simulink model "position_control_PD_with_Due"  (R2022a)
settings: Solver=FixedStepAuto  StartTime=0.0  StopTime=6  FixedStep=0.01  RelTol=1e-3  EnableMultiTasking=on
undefined symbols (not defined in the file or in its folder): a, b, kd2, kd4, kp2, kp4
libraries: arduinolib x11, arduinosensorlib x4
settings Model: SimulationMode=external  ExtModeTrigDuration=2  Creator=DCLab  LastModifiedBy=LabPC
settings OptimizationCC: EnhancedBackFolding=on  PassReuseOutputArgsAs=Individual arguments  ZeroExternalMemoryAtStartup=off  ZeroInternalMemoryAtStartup=off  MaxStackSize=64  OptimizeBlockOrder=speed  DifferentSizesBufferReuse=on  OptimizationCustomize=off  EfficientTunableParamExpr=on
settings DebuggingCC: ParameterTunabilityLossMsg=error  UnconnectedInputMsg=warning  UnconnectedOutputMsg=warning  UnconnectedLineMsg=warning
settings HardwareCC: ProdBitPerInt=16  ProdBitPerPointer=16  ProdBitPerSizeT=16  ProdBitPerPtrDiffT=16  ProdLargestAtomicFloat=None  ProdWordSize=8  ProdHWDeviceType=Atmel->AVR
settings SFSimCC: MATLABDynamicMemAlloc=off  SimTargetLang=C++
settings RTWCC: SystemTargetFile=ert.tlc  HardwareBoard=Arduino Uno  TemplateMakefile=ert_default_tmf  Toolchain=Arduino AVR  BuildConfiguration=Faster Runs  DLArmComputeVersion=19.05
settings CodeAppCC: ForceParamTrailComments=on  IgnoreCustomStorageClasses=off  OperatorAnnotations=on  SimulinkDataObjDesc=on  SFDataObjDesc=on  InsertBlockDesc=on
settings ERTTargetCC: SupportContinuousTime=on  SupportVariableSizeSignals=on  ExtMode=on  ExtModeTransport=3  ExtModeStaticAlloc=on  ExtModeStaticAllocSize=250  ExtModeMexFile=ext_xcp  ExtModeMexArgs=0 3 115200  ExtModeIntrfLevel=Level2 - Open

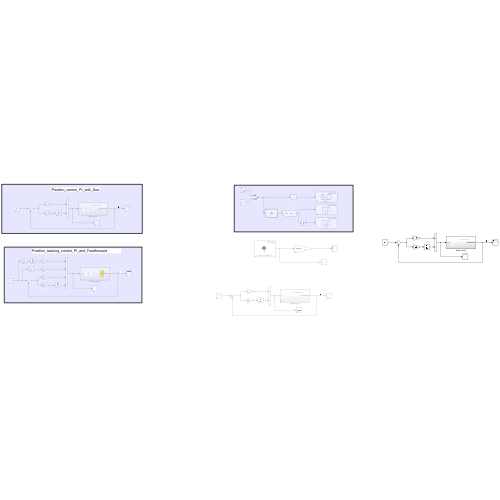
[thumbnail: Simulink's stored preview of the top-level diagram]
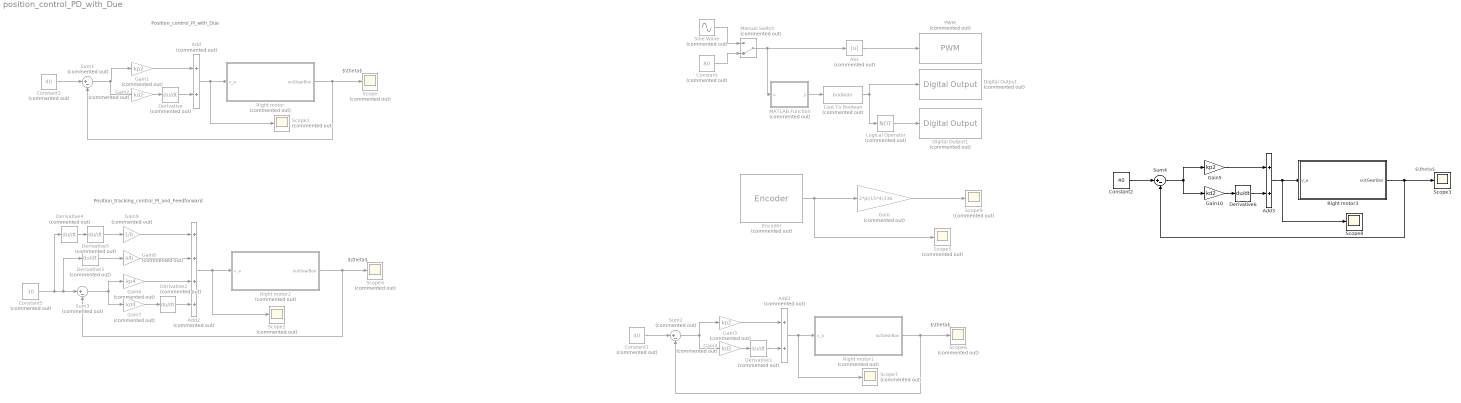
== system position_control_PD_with_Due ==
  note: Position_control_PI_with_Due
  note: $\theta$
  note: $\theta$
  note: Position_tracking_control_PI_and_Feedforward
  note: $\theta$
  note: $\theta$
  Abs : Abs  Commented=on  SaturateOnIntegerOverflow=off
  Add : Sum  Commented=on
  Add1 : Sum  Commented=on
  Add2 : Sum  Commented=on  Inputs=++++
  Add3 : Sum
  Cast To Boolean : DataTypeConversion  Commented=on  OutDataTypeStr=boolean  SaturateOnIntegerOverflow=off  RndMeth=Floor
  Constant : Constant  Commented=on  Value=80
  Constant1 : Constant  Commented=on  Value=40
  Constant2 : Constant  Value=40
  Constant3 : Constant  Commented=on  Value=40
  Constant5 : Constant  Commented=on  Value=30
  Derivative{,1..5} (6 alike) : Derivative  Commented=on
  Derivative6 : Derivative
  Digital Output : arduinolib/Digital Output  Commented=on  pinNumber=6  Direction=output  blockPlatform=arduino
  Digital Output1 : arduinolib/Digital Output  Commented=on  pinNumber=7  Direction=output  blockPlatform=arduino
  Encoder : arduinosensorlib/Encoder  Commented=on  InputA=2  InputB=3  Mode=Reset at each Sample time  SampleTime=-1
      settings: SourceProductBaseCode=ARDUINO
  Gain : Gain  Commented=on  Gain=2*pi/15*4/336
  Gain1 : Gain  Commented=on  Gain=kp2
  Gain10 : Gain  Gain=kd2
  Gain2 : Gain  Commented=on  Gain=kd2
  Gain3 : Gain  Commented=on  Gain=kp2
  Gain4 : Gain  Commented=on  Gain=kd2
  Gain5 : Gain  Gain=kp2
  Gain6 : Gain  Commented=on  Gain=kp4
  Gain7 : Gain  Commented=on  Gain=kd4
  Gain8 : Gain  Commented=on  Gain=a/b
  Gain9 : Gain  Commented=on  Gain=1/b
  Logical Operator : Logic  Commented=on  Operator=NOT  AllPortsSameDT=off  OutDataTypeStr=boolean
  MATLAB Function : MATLAB Function  Commented=on  TreatAsAtomicUnit=on
  Manual Switch : ManualSwitch  Commented=on  CurrentSetting=0
  PWM : arduinolib/PWM  Commented=on  pinNumber=5  frequencyType=Default  desiredFrequency=490.2  achievableFrequency=490.2
  Right motor : Subsystem  Commented=on
  Right motor1 : Subsystem  Commented=on
  Right motor2 : Subsystem  Commented=on
  Right motor3 : Subsystem
  Scope{,1..2,4..7,9} (8 alike) : Scope  Commented=on
  Scope3 : Scope
  Scope8 : Scope
  Sine Wave : Sin  Commented=on  Amplitude=255  SampleTime=0
  Sum1 : Sum  Commented=on  Inputs=|+-
  Sum2 : Sum  Commented=on  Inputs=|+-
  Sum3 : Sum  Commented=on  Inputs=|+-
  Sum4 : Sum  Inputs=|+-
  wires:
  Gain2/1 -> Derivative/1
  Sum1/1 -> Gain2/1, Gain1/1
  Derivative/1 -> Add/2
  Gain1/1 -> Add/1
  Add/1 -> Scope1/1, Right motor/1(v_a)
  Right motor/1(outGearBox) -> Sum1/2, Scope/1
  Constant3/1 -> Sum1/1
  Sum3/1 -> Gain6/1, Gain7/1
  Gain9/1 -> Add2/1
  Derivative2/1 -> Add2/4
  Gain6/1 -> Add2/3
  Constant5/1 -> Derivative4/1, Derivative3/1, Sum3/1
  Gain7/1 -> Derivative2/1
  Gain8/1 -> Add2/2
  Derivative3/1 -> Gain8/1
  Derivative4/1 -> Derivative5/1
  Derivative5/1 -> Gain9/1
  Right motor2/1(outGearBox) -> Sum3/2, Scope4/1
  Add2/1 -> Scope2/1, Right motor2/1(v_a)
  MATLAB Function/1(y) -> Cast To Boolean/1
  Cast To Boolean/1 -> Logical Operator/1, Digital Output/1
  Logical Operator/1 -> Digital Output1/1
  Abs/1 -> PWM/1
  Encoder/1 -> Scope5/1, Gain/1
  Sine Wave/1 -> Manual Switch/1
  Manual Switch/1 -> MATLAB Function/1(u), Abs/1
  Constant/1 -> Manual Switch/2
  Constant1/1 -> Sum2/1
  Right motor1/1(outGearBox) -> Scope6/1, Sum2/2
  Add1/1 -> Right motor1/1(v_a), Scope7/1
  Gain3/1 -> Add1/1
  Derivative1/1 -> Add1/2
  Sum2/1 -> Gain3/1, Gain4/1
  Gain4/1 -> Derivative1/1
  Constant2/1 -> Sum4/1
  Right motor3/1(outGearBox) -> Scope3/1, Sum4/2
  Add3/1 -> Right motor3/1(v_a), Scope8/1
  Gain5/1 -> Add3/1
  Derivative6/1 -> Add3/2
  Sum4/1 -> Gain5/1, Gain10/1
  Gain10/1 -> Derivative6/1
  Gain/1 -> Scope9/1

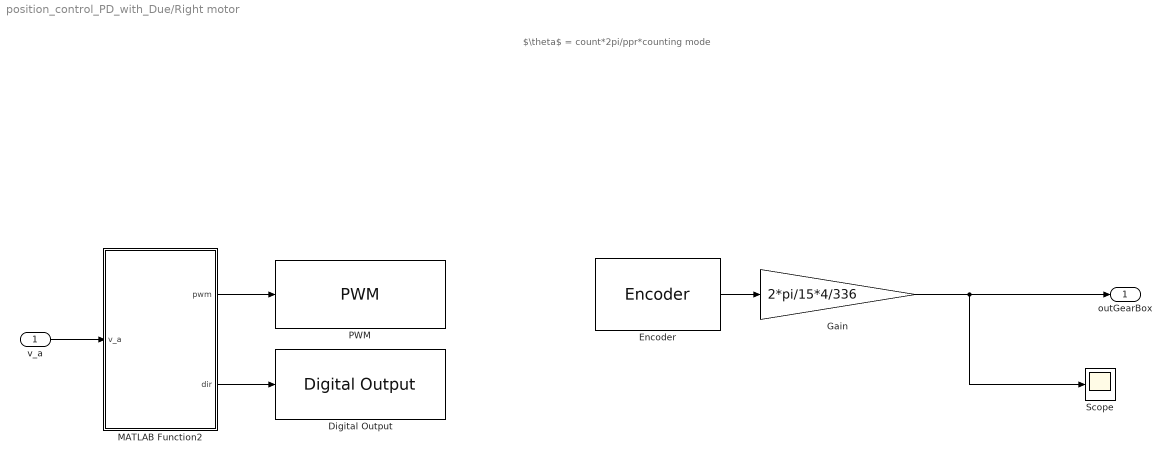
== system position_control_PD_with_Due/Right motor ==
  note: $\theta$ = count*2pi/ppr*counting mode
  v_a : Inport
  Digital Output : arduinolib/Digital Output  pinNumber=7  Direction=output  blockPlatform=arduino
  Encoder : arduinosensorlib/Encoder  InputA=2  InputB=3  Mode=No reset  SampleTime=-1
      settings: SourceProductBaseCode=ARDUINO
  Gain : Gain  Gain=2*pi/15*4/336
  MATLAB Function2 : MATLAB Function  TreatAsAtomicUnit=on
  PWM : arduinolib/PWM  pinNumber=5  frequencyType=Default  desiredFrequency=490.2  achievableFrequency=490.2
  Scope : Scope
  outGearBox : Outport
  wires:
  v_a/1 -> MATLAB Function2/1(v_a)
  MATLAB Function2/2(dir) -> Digital Output/1
  MATLAB Function2/1(pwm) -> PWM/1
  Encoder/1 -> Gain/1
  Gain/1 -> Scope/1, outGearBox/1

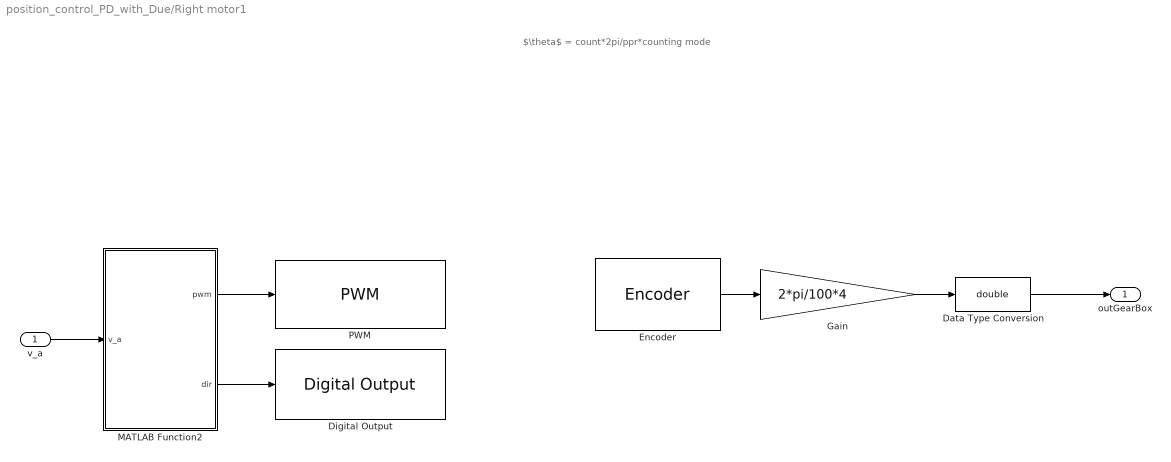
== system position_control_PD_with_Due/Right motor1 ==
  note: $\theta$ = count*2pi/ppr*counting mode
  v_a : Inport
  Data Type Conversion : DataTypeConversion  OutDataTypeStr=double  SaturateOnIntegerOverflow=off  RndMeth=Floor
  Digital Output : arduinolib/Digital Output  pinNumber=7  Direction=output  blockPlatform=arduino
  Encoder : arduinosensorlib/Encoder  InputA=2  InputB=3  Mode=No reset  SampleTime=-1
      settings: SourceProductBaseCode=ARDUINO
  Gain : Gain  Gain=2*pi/100*4
  MATLAB Function2 : MATLAB Function  TreatAsAtomicUnit=on
  PWM : arduinolib/PWM  pinNumber=6  frequencyType=Default  desiredFrequency=490.2  achievableFrequency=490.2
  outGearBox : Outport
  wires:
  Data Type Conversion/1 -> outGearBox/1
  Gain/1 -> Data Type Conversion/1
  Encoder/1 -> Gain/1
  MATLAB Function2/1(pwm) -> PWM/1
  MATLAB Function2/2(dir) -> Digital Output/1
  v_a/1 -> MATLAB Function2/1(v_a)

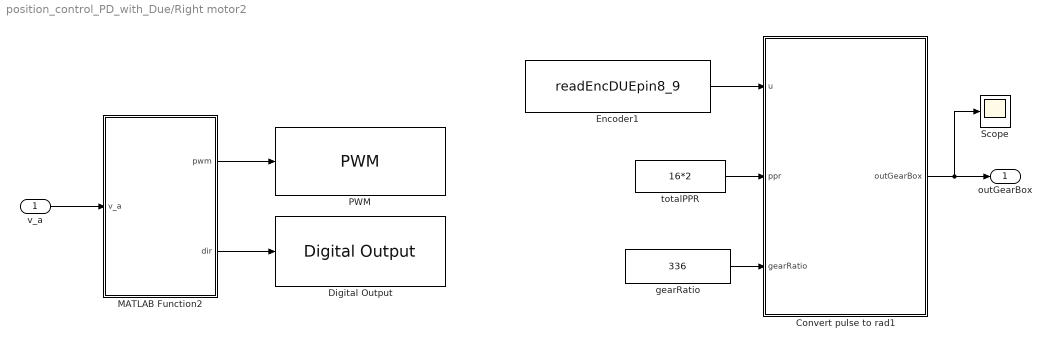
== system position_control_PD_with_Due/Right motor2 ==
  v_a : Inport
  Convert pulse to rad1 : MATLAB Function  TreatAsAtomicUnit=on
  Digital Output : arduinolib/Digital Output  pinNumber=7  Direction=output  blockPlatform=arduino
  Encoder1 : S-Function  InitFcn=try, set_param(gcb,'FunctionName','readEncDUEpin8_9'), end  FunctionName=readEncDUEpin8_9  SFunctionModules=readEncDUEpin8_9_wrapper  SFunctionDeploymentMode=off  EnableBusSupport=off  mask(S-Function Builder){}
      mask help: Simulink:masks:SFunctionBuilder_MD
      mask init:
      | val = [[.9  0.75 0.75 1 1 .9 .9 1]',[1 1 0.75 0.75 .9 .9 1 .9]'];try , sys = get_param(gcb,'SfunBuilderFcnName');if isempty(sys), sys = get_param(gcb,'FunctionName'); end,catch, sys = get_param(gcb,'FunctionName'); end
      settings: CopyFcn=set_param(gcbh,'LinkStatus','none')  PreSaveFcn=try, set_param(gcb,'FunctionName','readEncDUEpin8_9'), end  OpenFcn=sfunctionwizard(gcbh)
      mask Display:
      | plot(val(:,1),val(:,2))
      | disp(sys)
      | port_label('output',1,'count')
  MATLAB Function2 : MATLAB Function  TreatAsAtomicUnit=on
  PWM : arduinolib/PWM  pinNumber=5  frequencyType=Default  desiredFrequency=490.2  achievableFrequency=490.2
  Scope : Scope
  gearRatio : Constant  Value=336
  totalPPR : Constant  Value=16*2
  outGearBox : Outport
  wires:
  totalPPR/1 -> Convert pulse to rad1/2(ppr)
  v_a/1 -> MATLAB Function2/1(v_a)
  MATLAB Function2/2(dir) -> Digital Output/1
  MATLAB Function2/1(pwm) -> PWM/1
  gearRatio/1 -> Convert pulse to rad1/3(gearRatio)
  Convert pulse to rad1/1(outGearBox) -> Scope/1, outGearBox/1
  Encoder1/1 -> Convert pulse to rad1/1(u)

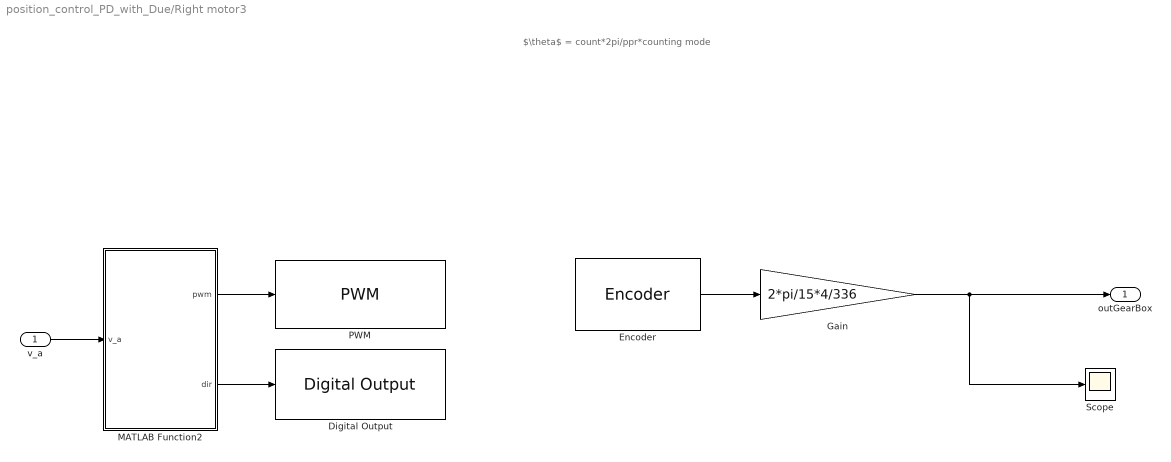
== system position_control_PD_with_Due/Right motor3 ==
  note: $\theta$ = count*2pi/ppr*counting mode
  v_a : Inport
  Digital Output : arduinolib/Digital Output  pinNumber=7  Direction=output  blockPlatform=arduino
  Encoder : arduinosensorlib/Encoder  InputA=2  InputB=3  Mode=No reset  SampleTime=-1
      settings: SourceProductBaseCode=ARDUINO
  Gain : Gain  Gain=2*pi/15*4/336
  MATLAB Function2 : MATLAB Function  TreatAsAtomicUnit=on
  PWM : arduinolib/PWM  pinNumber=5  frequencyType=Default  desiredFrequency=490.2  achievableFrequency=490.2
  Scope : Scope
  outGearBox : Outport
  wires:
  Gain/1 -> outGearBox/1, Scope/1
  Encoder/1 -> Gain/1
  MATLAB Function2/1(pwm) -> PWM/1
  MATLAB Function2/2(dir) -> Digital Output/1
  v_a/1 -> MATLAB Function2/1(v_a)

== matlab function position_control_PD_with_Due/Right motor1/MATLAB Function2 ==
  data: v_a input; pwm output; dir output
function [pwm,dir] = fcn(v_a)

vmax = 22.9;
pwm_cal = v_a*254/vmax;
if pwm_cal > 0
    pwm = pwm_cal;
    dir = 0;
elseif pwm_cal < 0
    pwm = abs(pwm_cal);
    dir = 1;
else
    pwm = 0;
    dir = 0;
end

== matlab function position_control_PD_with_Due/MATLAB Function ==
  data: u input; y output
function y = fcn(u)

y = (sign(u)+1)/2;

== matlab function position_control_PD_with_Due/Right motor2/Convert pulse to rad1 ==
  settings: updateMethod=DISCRETE
  data: u input; ppr input; gearRatio input; outGearBox output
function outGearBox = fcn(u,ppr,gearRatio)

persistent counter_num over_flag
if(isempty(counter_num)), counter_num = 0;end
if(isempty(over_flag)), over_flag = 0;end
pulse2radian = 2*pi/ppr; % 1 pulse = ?? radian

if(double(u) - counter_num > 40000), over_flag = over_flag-1;
elseif(double(u) - counter_num < -40000), over_flag = over_flag+1;
end

inGearBox = (double(u)+over_flag*(2^32 -1))*pulse2radian; 
outGearBox = inGearBox/gearRatio;
counter_num = double(u) ;

== matlab function position_control_PD_with_Due/Right motor2/MATLAB Function2 ==
  data: v_a input; pwm output; dir output
function [pwm,dir] = fcn(v_a)

vmax = 22.9;
%vmax = 10;
pwm_cal = v_a*254/vmax;
if pwm_cal > 0
    pwm = pwm_cal;
    dir = 0;
elseif pwm_cal < 0
    pwm = abs(pwm_cal);
    dir = 1;
else
    pwm = 0;
    dir = 0;
end

== matlab function position_control_PD_with_Due/Right motor3/MATLAB Function2 ==
  data: v_a input; pwm output; dir output
function [pwm,dir] = fcn(v_a)

vmax = 22.9;
pwm_cal = v_a*254/vmax;
if pwm_cal > 0
    pwm = pwm_cal;
    dir = 0;
elseif pwm_cal < 0
    pwm = abs(pwm_cal);
    dir = 1;
else
    pwm = 0;
    dir = 0;
end

== matlab function position_control_PD_with_Due/Right motor/MATLAB Function2 ==
  data: v_a input; pwm output; dir output
function [pwm,dir] = fcn(v_a)

vmax = 22.9;
pwm_cal = v_a*254/vmax;
if pwm_cal > 0
    pwm = pwm_cal;
    dir = 0;
elseif pwm_cal < 0
    pwm = abs(pwm_cal);
    dir = 1;
else
    pwm = 0;
    dir = 0;
end
